simulink model "gazeboExampleSimulink"  (R2017b)
settings: Solver=FixedStepDiscrete  StartTime=0.0  StopTime=inf  FixedStep=params.Ts  RelTol=1e-3  EnableMultiTasking=on
PreLoadFcn:
  | params = controlParamsGazebo;
  | 
  | rosshutdown;
  | loadIpAddresses;
  | rosinit(gazeboIp);
undefined symbols (not defined in the file): Angular, DiscIntNeverNeededParam, Linear
libraries: simulink x7, robotlib x4, visiontextngfix x1, visionsinks x1
settings Model: Creator=scastro  LastModifiedBy=scastro
settings SolverCC: PositivePriorityOrder=on
settings OptimizationCC: PassReuseOutputArgsAs=Individual arguments  MaxStackSize=64
settings DebuggingCC: ParameterTunabilityLossMsg=error
settings HardwareCC: ProdBitPerLong=64  ProdHWDeviceType=Intel->x86-64 (Linux 64)
settings RTWCC: SystemTargetFile=ert.tlc  HardwareBoard=Robot Operating System (ROS)  TemplateMakefile=ert_default_tmf  GenerateReport=on  Toolchain=Catkin  IncludeHyperlinkInReport=on  LaunchReport=on  TargetLang=C++  GenerateTraceInfo=on  GenerateTraceReport=on  GenerateTraceReportSl=on  GenerateTraceReportSf=on  GenerateTraceReportEml=on
settings CodeAppCC: ForceParamTrailComments=on  IgnoreCustomStorageClasses=off  OperatorAnnotations=on  SimulinkDataObjDesc=on  SFDataObjDesc=on  MATLABFcnDesc=on  InsertBlockDesc=on  StateflowObjectComments=on  MATLABSourceComments=on
settings ERTTargetCC: SupportVariableSizeSignals=on

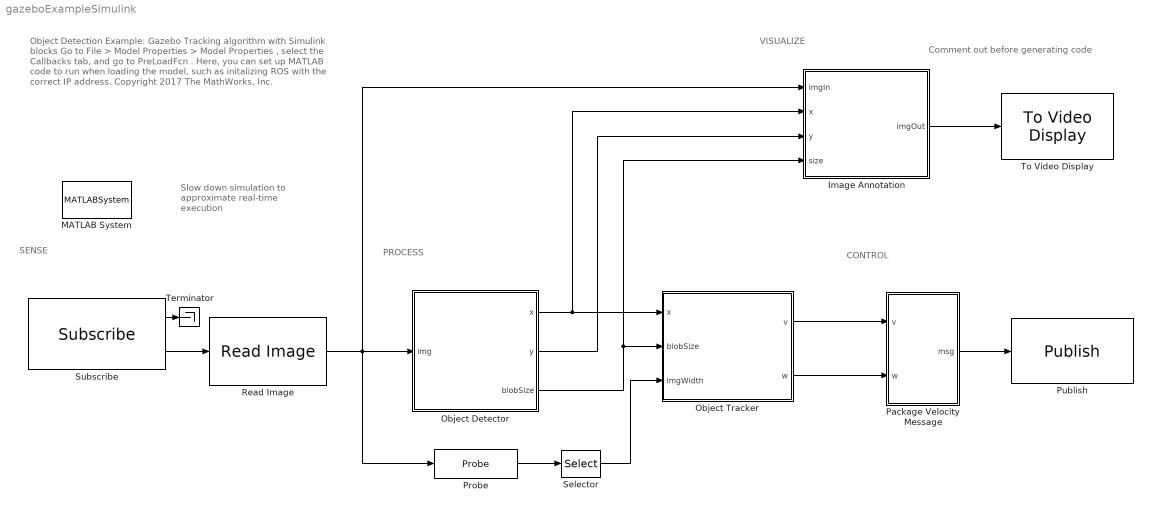
== system gazeboExampleSimulink ==
  note: Comment out before generating code
  note: CONTROL
  note: PROCESS
  note: SENSE
  note: VISUALIZE
  note: Slow down simulation to approximate real-time execution
  note: Object Detection Example: Gazebo
      | Tracking algorithm with Simulink blocks
      |
      | Go to File > Model Properties > Model Properties , select the Callbacks tab, and go to PreLoadFcn . Here, you can set up MATLAB code to run when loading the model, such as initalizing ROS with the correct IP address.
      |
      | Copyright 2017 The MathWorks, Inc.
  Image Annotation : Subsystem
  MATLAB System : MATLABSystem  System=ExampleHelperSimulationRateControl  SampleTime=0.02
      mask Type: ExampleHelperSimulationRateControl
      mask Display: disp('Rate Control');
  Object Detector : MATLAB Function  TreatAsAtomicUnit=on
  Object Tracker : Subsystem
  Package Velocity Message : Subsystem
  Probe : Probe  ProbeWidth=off  ProbeSampleTime=off  ProbeComplexSignal=off  ProbeSignalDimensions=on
  Publish : robotlib/Publish  SourceLibraryInfo=This block requires Robotics System Toolbox  topicSource=Select from ROS network  topic=/mobile_base/commands/velocity  messageType=geometry_msgs/Twist  messageQueueLength=1
      settings: SourceProductBaseCode=RO
  Read Image : robotlib/Read Image  SourceLibraryInfo=This block requires Robotics System Toolbox  MaximumImageSize=[480, 640]  ImageEncoding=rgb8  ShowAlphaOutput=off  ShowErrorCodeOutput=off  VariableSizeOutputs=off
      settings: SourceProductName=Robotics System Toolbox  SourceProductBaseCode=RO
  Selector : Selector  InputPortWidth=3  IndexOptions=Index vector (dialog)  Indices=2  OutputSizes=1
  Subscribe : robotlib/Subscribe  SourceLibraryInfo=This block requires Robotics System Toolbox  topicSource=Select from ROS network  topic=/camera/rgb/image_raw  messageType=sensor_msgs/Image  sampleTime=-1  messageQueueLength=1
      settings: SourceProductBaseCode=RO
  Terminator : Terminator
  To Video Display : visionsinks/To Video Display  windowSizeMode=Normal  openAtMdlStart=on  fullScreen=off  videoWindowX=653  videoWindowY=103  saveWindowSize=off  videoWindowWidth=699  videoWindowHeight=567  inputColorFormat=RGB  inputType=Obsolete  imagePorts=One multidimensional signal  OutputDevice=On-screen video monitor  dataOrg=Column-major  isWindowOpen=off
      settings: SourceProductName=Computer Vision System Toolbox
  wires:
  Object Detector/3(blobSize) -> Object Tracker/2(blobSize), Image Annotation/4(size)
  Object Detector/1(x) -> Object Tracker/1(x), Image Annotation/2(x)
  Image Annotation/1(imgOut) -> To Video Display/1
  Probe/1 -> Selector/1
  Selector/1 -> Object Tracker/3(imgWidth)
  Object Tracker/1(v) -> Package Velocity Message/1(v)
  Object Tracker/2(w) -> Package Velocity Message/2(w)
  Package Velocity Message/1(msg) -> Publish/1
  Subscribe/2 -> Read Image/1
  Object Detector/2(y) -> Image Annotation/3(y)
  Read Image/1 -> Object Detector/1(img), Image Annotation/1(imgIn), Probe/1
  Subscribe/1 -> Terminator/1

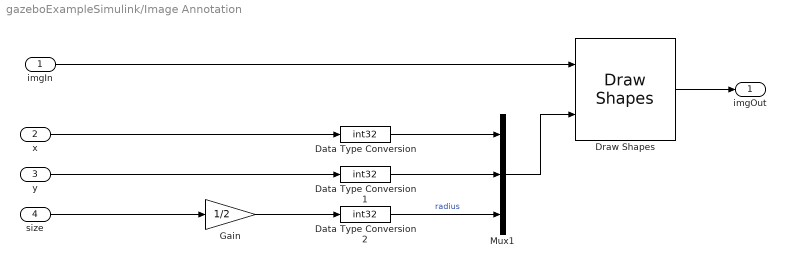
== system gazeboExampleSimulink/Image Annotation ==
  imgIn : Inport
  x : Inport  Port=2
  y : Inport  Port=3
  size : Inport  Port=4
  Data Type Conversion : DataTypeConversion  OutDataTypeStr=int32
  Data Type Conversion1 : DataTypeConversion  OutDataTypeStr=int32
  Data Type Conversion2 : DataTypeConversion  OutDataTypeStr=int32
  Draw Shapes : visiontextngfix/Draw Shapes  shape=Circles  fill=off  lineWidth=2  fillClrSource=Specify via dialog  display=User-specified value  intensity=200  color=[255 255 0]  opacity=0.6  viewport=Entire image  antialiasing=off  inType=Obsolete  imagePorts=One multidimensional signal  prodOutputMode=Binary point scaling  prodOutputWordLength=32  prodOutputFracLength=14  memoryMode=Specify word length  memoryWordLength=16  memoryFracLength=14  roundingMode=Floor  overflowMode=off
      settings: SourceProductName=Computer Vision System Toolbox
  Gain : Gain  Gain=1/2
  Mux1 : Mux  Inputs=3
  imgOut : Outport
  wires:
  y/1 -> Data Type Conversion1/1
  Data Type Conversion1/1 -> Mux1/2
  Data Type Conversion/1 -> Mux1/1
  x/1 -> Data Type Conversion/1
  imgIn/1 -> Draw Shapes/1
  Draw Shapes/1 -> imgOut/1
  Mux1/1 -> Draw Shapes/2
  Gain/1 -> Data Type Conversion2/1
  size/1 -> Gain/1
  Data Type Conversion2/1 -> Mux1/3  "radius"

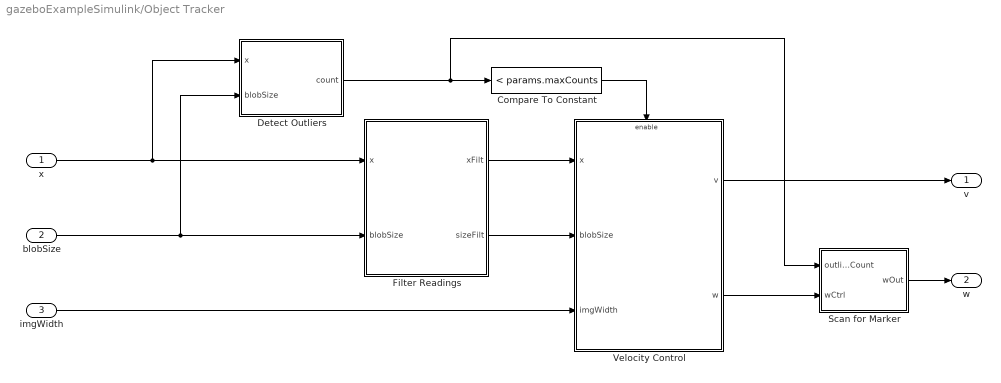
== system gazeboExampleSimulink/Object Tracker ==
  x : Inport
  blobSize : Inport  Port=2
  imgWidth : Inport  Port=3
  Compare To Constant : simulink/Logic and Bit Operations/Compare To Constant  relop=<  const=params.maxCounts  OutDataTypeStr=boolean
  Detect Outliers : Subsystem
  Filter Readings : Subsystem
  Scan for Marker : Subsystem
  Velocity Control : Subsystem
  v : Outport
  w : Outport  Port=2
  wires:
  blobSize/1 -> Filter Readings/2(blobSize), Detect Outliers/2(blobSize)
  Filter Readings/1(xFilt) -> Velocity Control/1(x)
  x/1 -> Filter Readings/1(x), Detect Outliers/1(x)
  Velocity Control/1(v) -> v/1
  imgWidth/1 -> Velocity Control/3(imgWidth)
  Detect Outliers/1(count) -> Compare To Constant/1, Scan for Marker/1(outlierCount)
  Filter Readings/2(sizeFilt) -> Velocity Control/2(blobSize)
  Compare To Constant/1 -> Velocity Control/Enable
  Velocity Control/2(w) -> Scan for Marker/2(wCtrl)
  Scan for Marker/1(wOut) -> w/1

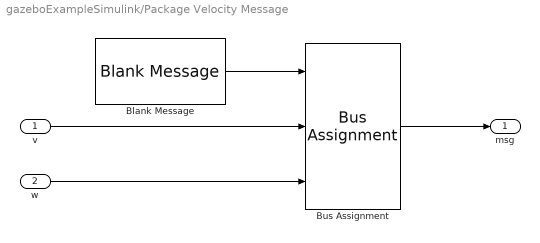
== system gazeboExampleSimulink/Package Velocity Message ==
  v : Inport
  w : Inport  Port=2
  Blank Message : robotlib/Blank Message  SourceLibraryInfo=This block requires Robotics System Toolbox  messageType=geometry_msgs/Twist  SampleTime=inf
      settings: SourceProductBaseCode=RO
  Bus Assignment : BusAssignment  AssignedSignals=Linear.X,Angular.Z
  msg : Outport
  wires:
  Blank Message/1 -> Bus Assignment/1
  Bus Assignment/1 -> msg/1
  w/1 -> Bus Assignment/3
  v/1 -> Bus Assignment/2

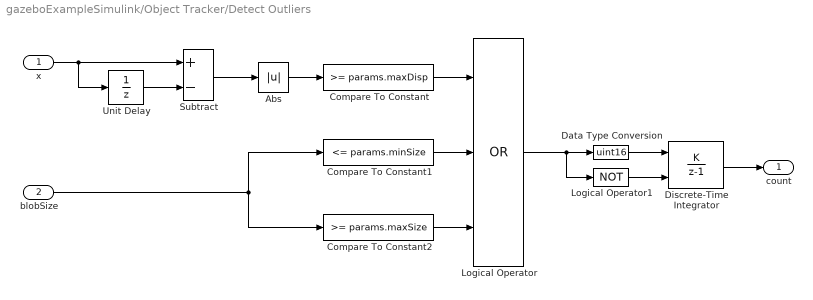
== system gazeboExampleSimulink/Object Tracker/Detect Outliers ==
  x : Inport
  blobSize : Inport  Port=2
  Abs : Abs
  Compare To Constant : simulink/Logic and Bit Operations/Compare To Constant  relop=>=  const=params.maxDisp  OutDataTypeStr=boolean
  Compare To Constant1 : simulink/Logic and Bit Operations/Compare To Constant  relop=<=  const=params.minSize  OutDataTypeStr=boolean
  Compare To Constant2 : simulink/Logic and Bit Operations/Compare To Constant  relop=>=  const=params.maxSize  OutDataTypeStr=boolean
  Data Type Conversion : DataTypeConversion  OutDataTypeStr=uint16
  Discrete-Time Integrator : DiscreteIntegrator  IntegratorMethod=Accumulation: Forward Euler  ExternalReset=level  InitialConditionSetting=State (most efficient)  SampleTime=-1  SaturateOnIntegerOverflow=on  LimitOutput=on  UpperSaturationLimit=1000  LowerSaturationLimit=0  ICPrevOutput=DiscIntNeverNeededParam  ICPrevScaledInput=DiscIntNeverNeededParam
  Logical Operator : Logic  Operator=OR  Inputs=3  AllPortsSameDT=off  OutDataTypeStr=boolean
  Logical Operator1 : Logic  Operator=NOT  AllPortsSameDT=off  OutDataTypeStr=boolean
  Subtract : Sum  Inputs=+-
  Unit Delay : UnitDelay  SampleTime=-1
  count : Outport
  wires:
  Compare To Constant2/1 -> Logical Operator/3
  blobSize/1 -> Compare To Constant2/1, Compare To Constant1/1
  Compare To Constant1/1 -> Logical Operator/2
  Compare To Constant/1 -> Logical Operator/1
  Abs/1 -> Compare To Constant/1
  Subtract/1 -> Abs/1
  Unit Delay/1 -> Subtract/2
  x/1 -> Unit Delay/1, Subtract/1
  Discrete-Time Integrator/1 -> count/1
  Data Type Conversion/1 -> Discrete-Time Integrator/1
  Logical Operator1/1 -> Discrete-Time Integrator/2
  Logical Operator/1 -> Logical Operator1/1, Data Type Conversion/1

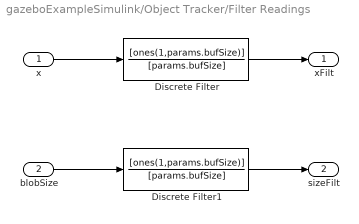
== system gazeboExampleSimulink/Object Tracker/Filter Readings ==
  x : Inport
  blobSize : Inport  Port=2
  Discrete Filter : DiscreteFilter  Numerator=[ones(1,params.bufSize)]  Denominator=[params.bufSize]
  Discrete Filter1 : DiscreteFilter  Numerator=[ones(1,params.bufSize)]  Denominator=[params.bufSize]
  xFilt : Outport
  sizeFilt : Outport  Port=2
  wires:
  Discrete Filter/1 -> xFilt/1
  Discrete Filter1/1 -> sizeFilt/1
  blobSize/1 -> Discrete Filter1/1
  x/1 -> Discrete Filter/1

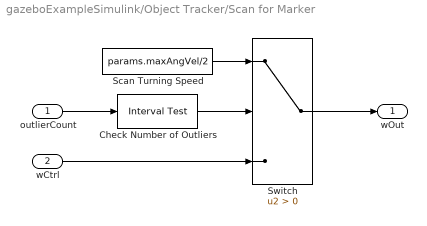
== system gazeboExampleSimulink/Object Tracker/Scan for Marker ==
  outlierCount : Inport
  wCtrl : Inport  Port=2
  Check Number of Outliers : simulink/Logic and Bit Operations/Interval Test  IntervalClosedRight=on  uplimit=500  IntervalClosedLeft=on  lowlimit=50  OutDataTypeStr=boolean
  Scan Turning Speed : Constant  Value=params.maxAngVel/2
  Switch : Switch  Criteria=u2 > Threshold
  wOut : Outport
  wires:
  wCtrl/1 -> Switch/3
  Scan Turning Speed/1 -> Switch/1
  Switch/1 -> wOut/1
  outlierCount/1 -> Check Number of Outliers/1
  Check Number of Outliers/1 -> Switch/2

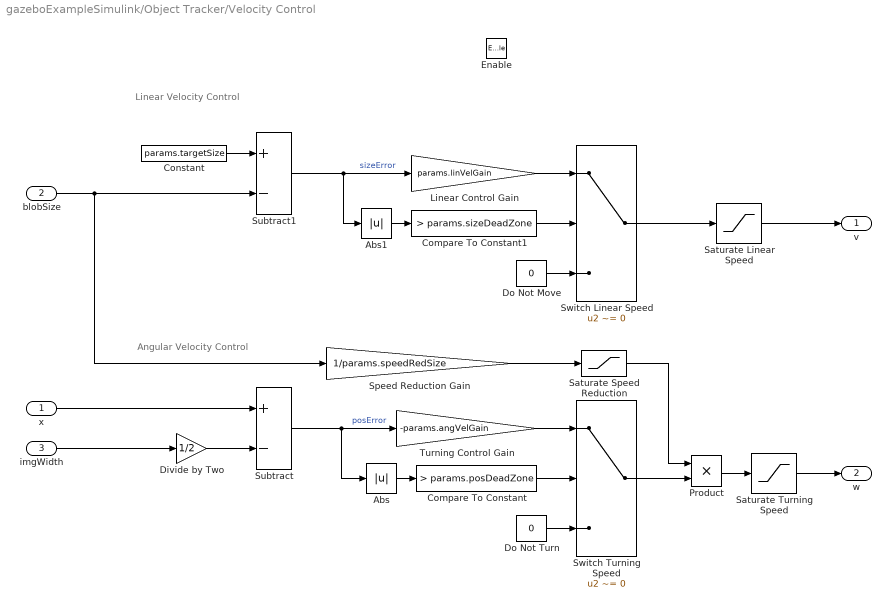
== system gazeboExampleSimulink/Object Tracker/Velocity Control ==
  note: Angular Velocity Control
  note: Linear Velocity Control
  x : Inport
  blobSize : Inport  Port=2
  imgWidth : Inport  Port=3
  Enable : EnablePort  StatesWhenEnabling=reset
  Abs : Abs
  Abs1 : Abs
  Compare To Constant : simulink/Logic and Bit Operations/Compare To Constant  relop=>  const=params.posDeadZone  OutDataTypeStr=boolean
  Compare To Constant1 : simulink/Logic and Bit Operations/Compare To Constant  relop=>  const=params.sizeDeadZone  OutDataTypeStr=boolean
  Constant : Constant  Value=params.targetSize
  Divide by Two : Gain  Gain=1/2
  Do Not Move : Constant  Value=0
  Do Not Turn : Constant  Value=0
  Linear Control Gain : Gain  Gain=params.linVelGain
  Product : Product
  Saturate Linear Speed : Saturate  UpperLimit=params.maxLinVel  LowerLimit=-params.maxLinVel
  Saturate Speed Reduction : Saturate  UpperLimit=1  LowerLimit=0
  Saturate Turning Speed : Saturate  UpperLimit=params.maxAngVel  LowerLimit=-params.maxAngVel
  Speed Reduction Gain : Gain  Gain=1/params.speedRedSize
  Subtract : Sum  Inputs=+-
  Subtract1 : Sum  Inputs=+-
  Switch Linear Speed : Switch  Criteria=u2 ~= 0
  Switch Turning Speed : Switch  Criteria=u2 ~= 0
  Turning Control Gain : Gain  Gain=-params.angVelGain
  v : Outport  OutputWhenDisabled=reset  InitialOutput=0
  w : Outport  Port=2  OutputWhenDisabled=reset  InitialOutput=0
  wires:
  x/1 -> Subtract/1
  imgWidth/1 -> Divide by Two/1
  Divide by Two/1 -> Subtract/2
  Subtract/1 -> Turning Control Gain/1, Abs/1  "posError"
  Turning Control Gain/1 -> Switch Turning Speed/1
  Abs/1 -> Compare To Constant/1
  Switch Turning Speed/1 -> Product/2
  Compare To Constant/1 -> Switch Turning Speed/2
  Do Not Turn/1 -> Switch Turning Speed/3
  Do Not Move/1 -> Switch Linear Speed/3
  Compare To Constant1/1 -> Switch Linear Speed/2
  Switch Linear Speed/1 -> Saturate Linear Speed/1
  Abs1/1 -> Compare To Constant1/1
  Linear Control Gain/1 -> Switch Linear Speed/1
  Subtract1/1 -> Linear Control Gain/1, Abs1/1  "sizeError"
  Constant/1 -> Subtract1/1
  Saturate Linear Speed/1 -> v/1
  Product/1 -> Saturate Turning Speed/1
  Speed Reduction Gain/1 -> Saturate Speed Reduction/1
  blobSize/1 -> Subtract1/2, Speed Reduction Gain/1
  Saturate Speed Reduction/1 -> Product/1
  Saturate Turning Speed/1 -> w/1

== matlab function gazeboExampleSimulink/Object Detector ==
  settings: updateMethod=DISCRETE
  data: x output; img input; y output; blobSize output
function [x,y,blobSize] = CircleDetection(img)
    
    % Initialize outputs
    x = 0;
    y = 0;
    blobSize = 0;
    
    % Call external function
    resizeScale = 0.5;
    [x,y,blobSize] = detectCircle(img,resizeScale);

end
